simulink model "QuadCopterSimple"  (R2014b)
settings: Solver=ode23t  StartTime=0.0  StopTime=10.0  MaxStep=0.0000001  RelTol=1e-7
undefined symbols (not defined in the file or in its folder): dc, g
libraries: Lib_Sensors x4, Lib_SimpleCopter x3
settings Model: Creator=Ehang  LastModifiedBy=Ehang
settings SolverCC: SolverResetMethod=Robust
settings ModelReferenceCC: ModelReferenceNumInstancesAllowed=Single

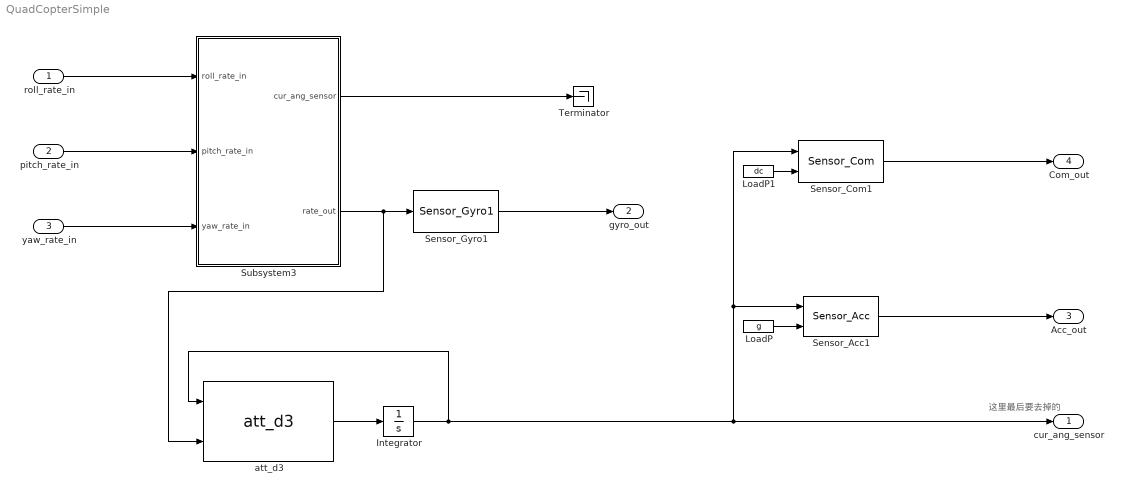
== system QuadCopterSimple ==
  note: 这里最后要去掉的
  roll_rate_in : Inport
  pitch_rate_in : Inport  Port=2
  yaw_rate_in : Inport  Port=3
  Integrator : Integrator  InitialCondition=[0;0;0]
  LoadP : Constant  Value=g  SampleTime=0
  LoadP1 : Constant  Value=dc  SampleTime=0
  Sensor_Acc1 : Lib_Sensors/Sensor_Acc
  Sensor_Com1 : Lib_Sensors/Sensor_Com
  Sensor_Gyro1 : Lib_Sensors/Sensor_Gyro1
  Subsystem3 : Subsystem
  Terminator : Terminator
  att_d3 : Lib_Sensors/att_d3
  cur_ang_sensor : Outport
  gyro_out : Outport  Port=2
  Acc_out : Outport  Port=3
  Com_out : Outport  Port=4
  wires:
  roll_rate_in/1 -> Subsystem3/1(roll_rate_in)
  Subsystem3/1(cur_ang_sensor) -> Terminator/1
  Subsystem3/2(rate_out) -> att_d3/2, Sensor_Gyro1/1
  pitch_rate_in/1 -> Subsystem3/2(pitch_rate_in)
  Integrator/1 -> att_d3/1, cur_ang_sensor/1, Sensor_Com1/1, Sensor_Acc1/1
  att_d3/1 -> Integrator/1
  LoadP/1 -> Sensor_Acc1/2
  Sensor_Acc1/1 -> Acc_out/1
  LoadP1/1 -> Sensor_Com1/2
  Sensor_Com1/1 -> Com_out/1
  yaw_rate_in/1 -> Subsystem3/3(yaw_rate_in)
  Sensor_Gyro1/1 -> gyro_out/1

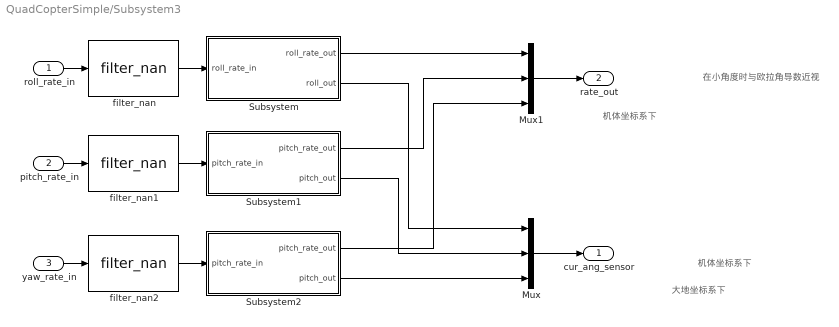
== system QuadCopterSimple/Subsystem3 ==
  note: 机体坐标系下
  note: 大地坐标系下
  note: 机体坐标系下
  note: 在小角度时与欧拉角导数近视
  roll_rate_in : Inport
  pitch_rate_in : Inport  Port=2
  yaw_rate_in : Inport  Port=3
  Mux : Mux  Inputs=3
  Mux1 : Mux  Inputs=3
  Subsystem : Subsystem
  Subsystem1 : Subsystem
  Subsystem2 : Subsystem
  filter_nan : Lib_SimpleCopter/filter_nan
  filter_nan1 : Lib_SimpleCopter/filter_nan
  filter_nan2 : Lib_SimpleCopter/filter_nan
  cur_ang_sensor : Outport
  rate_out : Outport  Port=2
  wires:
  roll_rate_in/1 -> filter_nan/1
  Subsystem/2(roll_out) -> Mux/1
  Subsystem/1(roll_rate_out) -> Mux1/1
  Mux1/1 -> rate_out/1
  Subsystem1/1(pitch_rate_out) -> Mux1/2
  Subsystem1/2(pitch_out) -> Mux/2
  yaw_rate_in/1 -> filter_nan2/1
  Subsystem2/1(pitch_rate_out) -> Mux1/3
  Subsystem2/2(pitch_out) -> Mux/3
  Mux/1 -> cur_ang_sensor/1
  pitch_rate_in/1 -> filter_nan1/1
  filter_nan/1 -> Subsystem/1(roll_rate_in)
  filter_nan1/1 -> Subsystem1/1(pitch_rate_in)
  filter_nan2/1 -> Subsystem2/1(pitch_rate_in)

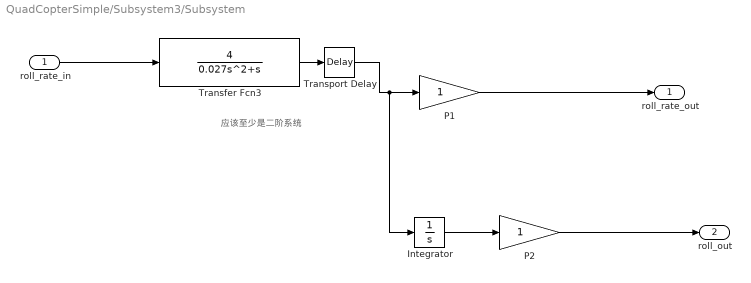
== system QuadCopterSimple/Subsystem3/Subsystem ==
  note: 应该至少是二阶系统
  roll_rate_in : Inport
  Integrator : Integrator
  P1 : Gain
  P2 : Gain
  Transfer Fcn3 : TransferFcn  Numerator=[4]  Denominator=[0.027 1 0]  AbsoluteTolerance=1e-19
  Transport Delay : TransportDelay  DelayTime=0.02606
  roll_rate_out : Outport
  roll_out : Outport  Port=2
  wires:
  roll_rate_in/1 -> Transfer Fcn3/1
  Integrator/1 -> P2/1
  Transfer Fcn3/1 -> Transport Delay/1
  P2/1 -> roll_out/1
  P1/1 -> roll_rate_out/1
  Transport Delay/1 -> P1/1, Integrator/1

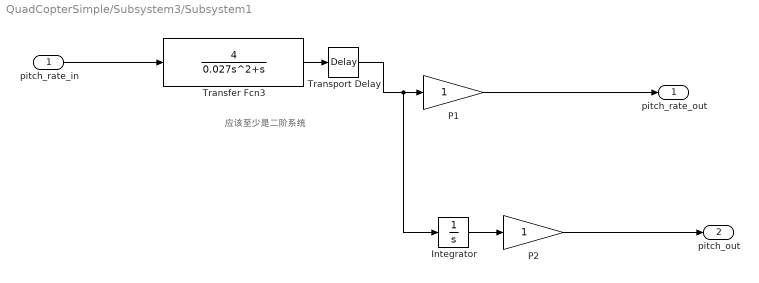
== system QuadCopterSimple/Subsystem3/Subsystem1 ==
  note: 应该至少是二阶系统
  pitch_rate_in : Inport
  Integrator : Integrator
  P1 : Gain
  P2 : Gain
  Transfer Fcn3 : TransferFcn  Numerator=[4]  Denominator=[0.027 1 0]  AbsoluteTolerance=1e-25
  Transport Delay : TransportDelay  DelayTime=0.02606
  pitch_rate_out : Outport
  pitch_out : Outport  Port=2
  wires:
  pitch_rate_in/1 -> Transfer Fcn3/1
  Integrator/1 -> P2/1
  Transfer Fcn3/1 -> Transport Delay/1
  P2/1 -> pitch_out/1
  P1/1 -> pitch_rate_out/1
  Transport Delay/1 -> P1/1, Integrator/1

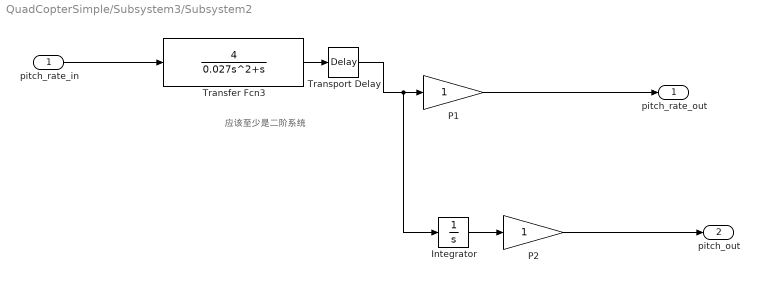
== system QuadCopterSimple/Subsystem3/Subsystem2 ==
  note: 应该至少是二阶系统
  pitch_rate_in : Inport
  Integrator : Integrator
  P1 : Gain
  P2 : Gain
  Transfer Fcn3 : TransferFcn  Numerator=[4]  Denominator=[0.027 1 0]  AbsoluteTolerance=1e-19
  Transport Delay : TransportDelay  DelayTime=0.02606
  pitch_rate_out : Outport
  pitch_out : Outport  Port=2
  wires:
  pitch_rate_in/1 -> Transfer Fcn3/1
  Integrator/1 -> P2/1
  Transfer Fcn3/1 -> Transport Delay/1
  P2/1 -> pitch_out/1
  P1/1 -> pitch_rate_out/1
  Transport Delay/1 -> P1/1, Integrator/1
